simulink model "VFlexP_small"  (R2026a)
settings: Solver=ode23tb  StopTime=2  FixedStep=5e-5
model workspace (MAT data in the model file):
  DCop_DCBUCK : object (value not decoded)
  Grid_CCVSC_idx = [2; 3; 4; 5; 6; 7; 8; 9; 10; 11; 12]
  Grid_CCVSCs = 1
  Grid_CCVSCs_buses = 1
  Grid_CCVSCs_toM = [0 1 0 0 0 0 0 0 0 0 0 0 ... (781 elements, 71x11)]
  Grid_C_Lines = 0
  Grid_Cbuses = [0.00666666666667 0.00666666666667]
  Grid_DC : object (value not decoded)
  Grid_DCop_DCBUCK : object (value not decoded)
  Grid_DCop_DC_PES : object (value not decoded)
  Grid_DFIGs = 1
  Grid_DFIGs_buses = 1
  Grid_DGs : string (value not decoded)
  Grid_From_buses = 1
  Grid_GFls = 1
  Grid_GFls_buses = 1
  Grid_GFr_idx = 1
  Grid_GFrs = 1
  Grid_GFrs_buses = 1
  Grid_GFrs_toM = [1; 0]
  Grid_IG_idx = 1
  Grid_IGs = 1
  Grid_IGs_buses = 1
  Grid_IGs_toM = [1; 0; 0]
  Grid_L_Lines = 0.05
  Grid_L_Loads = [0 0]
  Grid_Lines_fromM : object (value not decoded)
  Grid_Lines_toM : object (value not decoded)
  Grid_Load_buses = [1; 2]
  Grid_Load_busesDC = []
  Grid_MSGs = 1
  Grid_MSGs_buses = 1
  Grid_Nbuses = 2
  Grid_PQ_gen = 3
  Grid_Ploads = [0.0075 0.0075]
  Grid_PloadsDC = []
  Grid_Ps_lf = 0.51232912
  Grid_Qloads = [0 0]
  Grid_Qs_lf = -0.00723209333333
  Grid_R_Lines = 0.005
  Grid_R_Loads = [2 2]
  Grid_R_Loads_DC = 0
  Grid_Rcf = [150 150]
  Grid_SCs = 1
  Grid_SCs_buses = 1
  Grid_SG_idx = 1
  Grid_SGs = 1
  Grid_SGs_buses = 1
  Grid_SGs_toM = [1; 0]
  Grid_To_buses = 2
  Grid_VCVSC_idx = [1; 2; 3; 4; 5; 6; 7; 8; 9; 10; 11; 12]
  Grid_VCVSCs = 1
  Grid_VCVSCs_buses = [1; 2; 3; 6; 8; 9; 12; 58; 59; 60; 63; 65]
  Grid_VCVSCs_toM = [1 0 0 0 0 0 0 0 0 0 0 0 ... (852 elements, 71x12)]
  Grid_VSM_idx = 2
  Grid_VSMs = 1
  Grid_VSMs_buses = 1
  Grid_VSMs_toM = [0; 1]
  Grid_admitt_matrix = [2.15353135314-19.7953135314i  -1.9801980198+19.801980198i; -1.9801980198+19.801980198i  2.15353135314-19.7953135314i]
  Grid_admitt_matrix_noloads = [1.98686468647-19.7953135314i  -1.9801980198+19.801980198i; -1.9801980198+19.801980198i  1.98686468647-19.7953135314i]
  Grid_bus = [1; 2]
  Grid_busDC_complexity = 1
  Grid_busDC_complexity_PF = 2
  Grid_bus_complexity = [1 1]
  Grid_bus_complexity_PF = [1 1]
  Grid_buses_lf = 1
  Grid_conductance_matrix = 0.00666666666667
  Grid_conductance_matrix_noloads = 0.00666666666667
  Grid_fref : object (value not decoded)
  Grid_gen_static_params : mBase (value not decoded)
  Grid_iPs_lf = 1.95187031336
  Grid_iQs_lf = -138.272551792
  Grid_iadmitt_matrix = [2.88165849328-0.0982918688642i  2.87905051706-0.123273862303i; 2.87905051706-0.123273862303i  2.88165849328-0.0982918688642i]
  Grid_iadmitt_matrix_noloads = [37.5012524798-37.4874983544i  37.4987475202-37.5125016456i; 37.4987475202-37.5125016456i  37.5012524798-37.4874983544i]
  Grid_iconductance_matrix = 150
  Grid_iconductance_matrix_noloads = 150
  Grid_init_OK_bool = 1
  Grid_intconv_PF : object (value not decoded)
  Grid_lf_op : op_report (value not decoded)
  Grid_lineDC_complexity = []
  Grid_lineDC_complexity_PF = []
  Grid_line_complexity = 1
  Grid_line_complexity_PF = 3
  Grid_loadDC_complexity = []
  Grid_loadDC_complexity_PF = []
  Grid_load_complexity = [3 3]
  Grid_load_complexity_PF = [4 4]
  Grid_opDC_CCVSC : object (value not decoded)
  Grid_opDC_VSM : object (value not decoded)
  Grid_opGFr : object (value not decoded)
  Grid_opVCVSC : object (value not decoded)
  Grid_op_CCVSC : object (value not decoded)
  Grid_op_IG : object (value not decoded)
  Grid_op_SG : object (value not decoded)
  Grid_op_VSM : object (value not decoded)
  Grid_shift_lines = 0
  Grid_tap_lines = 1
  Grid_v_buses_mod = [1 1]
  LinsysParamChangeStruct : Param1 (value not decoded)
  Lline = 0.01
  Rline = 1e-05
  linsys : object (value not decoded)
values from neighbouring files (symbols this model uses):
  block_idx = evalin(mdlWks, [bvarname Generators{i} '_idx'])    [fun_init_units_callback.m]
  Fb = areas    [fun_MATPOWER_to_Excel.m]
  Fi = evalin('base', get_param(block, 'Fi'))    [fun_init_GFr.m]    (also in fun_init_intconv_DC_VSM.m)
  Lf = evalin('base', get_param(block, 'Lf'))    [fun_init_GFr.m]    (also in fun_init_intconv_DC_VSM.m)
  Rf = evalin('base', get_param(block, 'Rf'))    [fun_init_GFr.m]    (also in fun_init_intconv_DC_VSM.m)
symbols that are objects in the model workspace (value not decoded): Grid_DCop_DC_PES, Grid_DCop_DCBUCK, Grid_op_CCVSC, Grid_op_IG, Grid_op_SG, Grid_op_VSM, Grid_opDC_CCVSC, Grid_opDC_VSM, Grid_opGFr, Grid_opVCVSC
undefined symbols (not defined in the file or in its folder): block_buses_DC, CCVSC_idx, Cf, costs, costs2, DFIGs_nodes, DiscIntNeverNeededParam, entity, From_nodes, grid_linsys, Grid_op_DFIG, Grid_op_DFIG_PQ, Grid_op_MSG, Grid_op_SC, Grid_op_VCVSC, Hv, initial_states_grid, Kic, Kiv, Kp_theta, Kp_w, Kpc, Kpv, last_send, Lc, m, Matrix_flux_to_i, mD, mp, MSGs_buses, Nbuses_DC, nq, op_VCVSC, Psche, Rc, rkq1, rkq2, SCs_buses, SCs_nodes, sec_control_structure, set_asked, set_DG_up, set_extra_satur, set_sending_cost, SGs_buses, SGs_nodes, Tf, To_nodes, VI_L, VI_R, WOF_Tf, xkq1, xkq2
libraries: simulink x1045, eeGeneralControl x12, eeTransforms x1, sl_discontinuities x1
(part 8 of 50)

== system VFlexP_small/Grid/Dynamic/Secondary Control/Matrices1 ==
  tertiary_refs : Inport
  start_SC : Inport  Port=2
  elec : Inport  Port=3
  Assignment{,1..2,13} (4 alike) : Assignment  NumberOfDimensions=2  DiagnosticForDimensions=Warning  IndexOptions=Index vector (dialog),Assign all  Indices=2,1  OutputSizes=1,1
  Assignment10 : Assignment  NumberOfDimensions=2  DiagnosticForDimensions=Warning  IndexOptions=Index vector (dialog),Assign all  Indices=1,1  OutputSizes=1,1
  Assignment{3..4,9,11} (4 alike) : Assignment  DiagnosticForDimensions=Warning  IndexOptions=Index vector (port)  Indices=1  OutputSizes=1
  Assignment12 : Assignment  NumberOfDimensions=2  DiagnosticForDimensions=Warning  IndexOptions=Index vector (dialog),Assign all  Indices=1,1  OutputSizes=1,1
  Assignment{5..8} (4 alike) : Assignment  NumberOfDimensions=2  DiagnosticForDimensions=Warning  IndexOptions=Index vector (port),Assign all  Indices=1,1  OutputSizes=1,1
  Cast To Double1 : DataTypeConversion  OutDataTypeStr=double  SaturateOnIntegerOverflow=off  RndMeth=Floor
  Compare To Constant : simulink/Logic and Bit Operations/Compare To Constant  relop=>  const=0.8  OutDataTypeStr=boolean
  Compare To Constant1 : simulink/Logic and Bit Operations/Compare To Constant  relop=<  const=0  OutDataTypeStr=boolean
  Compare To Constant2 : simulink/Logic and Bit Operations/Compare To Constant  relop=>  const=3  OutDataTypeStr=boolean
  Constant : Constant  Commented=on  Value=costs'  VectorParams1D=off
  Constant1 : Constant  Commented=on  Value=2*costs2'  VectorParams1D=off
  Constant10 : Constant  Value=A_P_sc  VectorParams1D=off
  Constant11 : Constant  Value=A_v_sc  VectorParams1D=off
  Constant12 : Constant  Value=A_Q_sc  VectorParams1D=off
  Constant13 : Constant
  Constant14 : Constant  Value=0
  Constant15 : Constant  Value=zeros(1, length(buses_lf))  VectorParams1D=off
  Constant16 : Constant  Commented=on  Value=sec_control_structure
  Constant18 : Constant  Commented=on  Value=sec_control_structure
  Constant19 : Constant  Commented=on  VectorParams1D=off
  Constant2 : Constant  Value=repmat([1 1 1 1]', 1, length(buses_lf))
  Constant20 : Constant  Value=passM  VectorParams1D=off
  Constant3 : Constant  Commented=on
  Constant4 : Constant  Value=length(buses_lf)
  Constant5 : Constant  Value=g_f_sc'  VectorParams1D=off
  Constant6 : Constant  Value=g_P_sc'  VectorParams1D=off
  Constant7 : Constant  Value=g_v_sc'  VectorParams1D=off
  Constant8 : Constant  Value=g_Q_sc'  VectorParams1D=off
  Constant9 : Constant  Value=A_f_sc  VectorParams1D=off
  Display{,1..9} (10 alike) : Display
  Divide : Product  Commented=on  Inputs=*/
  Gain1 : Gain  Commented=on  Gain=1/400
  Gain11 : Gain  Commented=on  Gain=1/400
  Gain2 : Gain  Gain=20
  Gain9 : Gain  Gain=-1
  Integrator : Integrator
  Integrator1 : Integrator  ExternalReset=rising
  Matrix Concatenate : Concatenate  NumInputs=4  Mode=Multidimensional array
  Matrix Concatenate1 : Concatenate  NumInputs=3  Mode=Multidimensional array
  Matrix Concatenate2 : Concatenate  NumInputs=4  Mode=Multidimensional array
  Matrix Multiply{,1..4} (5 alike) : Product  Multiplication=Matrix(*)
  Memory1 : Memory
  Memory2 : Memory  InitialCondition=1
  Mod : Math  Operator=mod
  Multiport Switch : MultiPortSwitch  Commented=on  Inputs=5  SaturateOnIntegerOverflow=off  InputSameDT=off
  NOT : Logic  Operator=NOT  IconShape=distinctive  AllPortsSameDT=off  OutDataTypeStr=boolean
  OR1 : Logic  Operator=OR  Inputs=3  IconShape=distinctive  AllPortsSameDT=off  OutDataTypeStr=boolean
  One : Constant  OutDataTypeStr=Inherit: Inherit via back propagation
  One1 : Constant  OutDataTypeStr=Inherit: Inherit via back propagation
  One3 : Constant  Commented=on  OutDataTypeStr=Inherit: Inherit via back propagation
  Product{,2..4,7,9..12} (9 alike) : Product
  Product1 : Product  Commented=on
  Product13 : Product  Commented=on
  Product14 : Product  Commented=on
  Relational Operator : RelationalOperator  Operator===  OutDataTypeStr=boolean  RndMeth=Simplest  InputSameDT=off
  Relational Operator1 : RelationalOperator  Operator===  OutDataTypeStr=boolean  RndMeth=Simplest  InputSameDT=off
  Selector{,9,19,22,26,28} (6 alike) : Selector  NumberOfDimensions=2  InputPortWidth=3  IndexOptions=Index vector (dialog),Select all  Indices=1,1  OutputSizes=1,1
  Selector{1,7,10,13..15,20..21,23..25,27} (12 alike) : Selector  NumberOfDimensions=2  InputPortWidth=3  IndexOptions=Index vector (dialog),Select all  Indices=2,1  OutputSizes=1,1
  Selector11 : Selector  NumberOfDimensions=2  InputPortWidth=3  IndexOptions=Index vector (dialog),Select all  Indices=4,1  OutputSizes=1,1
  Selector12 : Selector  NumberOfDimensions=2  InputPortWidth=length(buses_lf)  IndexOptions=Index vector (dialog),Index vector (port)  Indices=6,1  OutputSizes=1,1
  Selector16 : Selector  NumberOfDimensions=2  InputPortWidth=length(buses_lf)  IndexOptions=Index vector (dialog),Index vector (port)  Indices=2,1  OutputSizes=1,1
  Selector17 : Selector  NumberOfDimensions=2  InputPortWidth=3  IndexOptions=Index vector (dialog),Index vector (port)  Indices=1,1  OutputSizes=1,1
  Selector18 : Selector  Commented=on  NumberOfDimensions=2  InputPortWidth=3  IndexOptions=Index vector (dialog),Select all  Indices=2,1  OutputSizes=1,1
  Selector2 : Selector  NumberOfDimensions=2  InputPortWidth=3  IndexOptions=Index vector (dialog),Select all  Indices=3,1  OutputSizes=1,1
  Selector3 : Selector  NumberOfDimensions=2  InputPortWidth=3  IndexOptions=Index vector (dialog),Select all  Indices=4,1  OutputSizes=1,1
  Selector4 : Selector  NumberOfDimensions=2  InputPortWidth=3  IndexOptions=Index vector (dialog),Select all  Indices=5,1  OutputSizes=1,1
  Selector5 : Selector  NumberOfDimensions=2  InputPortWidth=3  IndexOptions=Index vector (dialog),Select all  Indices=6,1  OutputSizes=1,1
  Selector6 : Selector  NumberOfDimensions=2  InputPortWidth=3  IndexOptions=Index vector (dialog),Select all  Indices=1:4,1  OutputSizes=1,1
  Selector8 : Selector  NumberOfDimensions=2  InputPortWidth=3  IndexOptions=Index vector (dialog),Select all  Indices=3,1  OutputSizes=1,1
  Sum{,1..3,5,9,11} (7 alike) : Sum  Inputs=|++
  Sum of Elements{,1..3} (4 alike) : Sum  Inputs=+  CollapseMode=Specified dimension  CollapseDim=2
  Sum10 : Sum  Inputs=|+-
  Sum4 : Sum  Inputs=|-+
  Sum6 : Sum  Inputs=|+-
  Sum7 : Sum  Commented=on  Inputs=|++
  Switch : Switch  Criteria=u2 > Threshold  SaturateOnIntegerOverflow=off  InputSameDT=off
  Switch1 : Switch  Criteria=u2 > Threshold  SaturateOnIntegerOverflow=off  InputSameDT=off
  Switch2 : Switch  Commented=on  Criteria=u2 > Threshold  SaturateOnIntegerOverflow=off  InputSameDT=off
  Switch3 : Switch  Commented=on  Criteria=u2 > Threshold  Threshold=1  SaturateOnIntegerOverflow=off  InputSameDT=off
  Transport Delay : TransportDelay  DelayTime=0.1  PadeOrder=3
  Transpose{,1..17} (18 alike) : Math  Operator=transpose
  Triggered Subsystem : Subsystem  TreatAsAtomicUnit=on
  Zero : Constant  Value=zeros(1, length(buses_lf))  VectorParams1D=off  OutDataTypeStr=Inherit: Inherit via back propagation
  Zero1 : Constant  Value=zeros(1, length(buses_lf))  VectorParams1D=off  OutDataTypeStr=Inherit: Inherit via back propagation
  Zero2 : Constant  Value=zeros(1, length(buses_lf))  VectorParams1D=off  OutDataTypeStr=Inherit: Inherit via back propagation
  saturation_P : Subsystem
  saturation_P2 : Subsystem
  start_SC1 : InportShadow  Port=2
  secondary_refs : Outport
  wires:
  Selector3/1 -> Transpose3/1  "Q"
  Selector/1 -> Transpose/1  "f"
  Selector1/1 -> Product2/1, Transpose13/1  "P"
  Selector2/1 -> Transpose2/1  "v"
  Sum/1 -> Transpose4/1
  Product9/1 -> Sum/2
  Product10/1 -> Sum1/2
  Matrix Multiply2/1 -> Sum2/1
  Product11/1 -> Sum2/2
  Product12/1 -> Sum3/2
  Sum2/1 -> Transpose6/1
  Sum3/1 -> Transpose7/1
  Matrix Multiply3/1 -> Sum3/1
  Transpose/1 -> Matrix Multiply/2
  Transpose1/1 -> Matrix Multiply1/2
  Transpose2/1 -> Matrix Multiply2/2
  Transpose3/1 -> Matrix Multiply3/2
  Transpose6/1 -> Matrix Concatenate/3
  Transpose7/1 -> Matrix Concatenate/4
  Selector8/1 -> Transpose10/1
  Selector4/1 -> Matrix Concatenate1/2
  start_SC/1 -> Switch/2
  Switch/1 -> secondary_refs/1, Selector19/1, Selector15/1
  Selector5/1 -> Matrix Concatenate1/3
  Selector9/1 -> Transpose8/1
  Selector10/1 -> Transpose9/1
  Selector11/1 -> Transpose11/1
  Sum5/1 -> Switch/1
  Transpose8/1 -> Product9/2
  Transpose9/1 -> Product10/2
  Transpose10/1 -> Product11/2
  Transpose11/1 -> Product12/2
  Matrix Concatenate/1 -> Sum6/1
  start_SC1/1 -> Product/2
  Transport Delay/1 -> Selector2/1, Selector3/1, Selector1/1, Selector/1, Gain9/1
  Constant1/1 -> Product1/1
  Product2/1 -> Transpose1/1
  [gaincost] -> Product2/2
  Product7/1 -> Assignment/1, Selector7/1
  [gaincost] -> Product3/2
  Selector7/1 -> Product3/1
  Assignment/1 -> Sum6/2, Selector24/1
  saturation_P/1(out) -> Matrix Concatenate/2, Relational Operator/1
  Product3/1 -> Assignment/2
  Selector13/1 -> [Pref]
  Selector14/1 -> Switch2/2, Switch1/1
  Switch1/1 -> Assignment2/2
  Transpose4/1 -> Matrix Concatenate/1
  Matrix Multiply1/1 -> Sum1/1
  Matrix Multiply/1 -> Sum/1
  Sum of Elements/1 -> Transpose14/1
  Sum of Elements1/1 -> Transpose15/1
  Sum of Elements2/1 -> Transpose16/1
  Sum of Elements3/1 -> Transpose17/1
  Transpose17/1 -> Matrix Concatenate2/4
  Transpose16/1 -> Matrix Concatenate2/3
  Transpose14/1 -> Matrix Concatenate2/2
  Transpose15/1 -> Matrix Concatenate2/1
  Selector6/1 -> Product7/1
  Matrix Concatenate2/1 -> Product7/2
  [A_f_sc] -> Sum of Elements1/1
  [A_P_sc] -> Sum of Elements/1
  [A_Q_sc] -> Sum of Elements3/1
  [A_v_sc] -> Sum of Elements2/1
  [A_f_sc] -> Matrix Multiply/1
  [A_P_sc] -> Matrix Multiply1/1
  [A_v_sc] -> Matrix Multiply2/1
  [A_Q_sc] -> Matrix Multiply3/1
  [g_f_sc] -> Product9/1
  [g_v_sc] -> Product11/1
  [g_Q_sc] -> Product12/1
  [g_P_sc] -> Product10/1
  Constant5/1 -> Assignment3/1
  Constant13/1 -> Assignment4/2, Assignment3/2
  [leader] -> Assignment4/3, Assignment3/3
  Constant6/1 -> [g_P_sc]
  Constant8/1 -> [g_Q_sc]
  Constant7/1 -> Assignment4/1
  Constant9/1 -> Assignment5/1
  Constant12/1 -> Assignment8/1
  Constant11/1 -> Assignment7/1
  Constant10/1 -> Assignment6/1
  [leader] -> Assignment9/3
  [leader] -> Assignment5/3, Assignment6/3, Assignment7/3, Assignment8/3
  Constant14/1 -> Assignment9/2
  Zero/1 -> Assignment9/1
  Assignment9/1 -> Assignment8/2, Assignment6/2
  Zero1/1 -> Assignment7/2, Assignment5/2
  Memory2/1 -> Selector12/2, Sum10/1, Selector16/2
  elec/1 -> Selector18/1, Selector12/1, Selector16/1, Sum4/2
  Selector16/1 -> Compare To Constant1/1, Compare To Constant/1
  Cast To Double1/1 -> Integrator1/1
  Mod/1 -> Sum9/1
  One/1 -> Sum9/2
  Triggered Subsystem/1(Out1) -> Mod/1
  Constant4/1 -> Mod/2
  [leader] -> Memory2/1
  Compare To Constant/1 -> OR1/1
  Compare To Constant1/1 -> OR1/2
  [leader] -> Assignment11/3, Selector17/2
  Selector17/1 -> Assignment11/2
  Constant15/1 -> Assignment11/1
  Integrator1/1 -> Compare To Constant2/1
  Compare To Constant2/1 -> Memory1/1, Triggered Subsystem/Trigger
  OR1/1 -> Cast To Double1/1
  Memory1/1 -> Integrator1/2
  Sum7/1 -> Gain11/1
  Gain11/1 -> Multiport Switch/5, Product13/2, Product13/1
  Product1/1 -> Sum7/2
  Selector18/1 -> Product1/2
  Constant3/1 -> [gaincost], Multiport Switch/2
  Constant16/1 -> Multiport Switch/1
  Sum10/1 -> Triggered Subsystem/1(In1)
  One1/1 -> Sum10/2
  Matrix Concatenate1/1 -> Sum5/1
  Constant/1 -> Gain1/1, Sum7/1
  Gain1/1 -> Multiport Switch/3, Product14/2, Product14/1
  Product14/1 -> Multiport Switch/4
  Product13/1 -> Multiport Switch/6
  Multiport Switch/1 -> Divide/2, Switch2/1
  Constant18/1 -> Switch3/2
  Divide/1 -> Switch3/1
  One3/1 -> Switch3/3
  Constant19/1 -> Divide/1
  tertiary_refs/1 -> Sum4/1, Selector13/1, Selector4/1, Selector5/1, Switch/3, Sum5/2
  Constant20/1 -> Matrix Multiply4/1
  Matrix Multiply4/1 -> Transpose12/1
  [awup1] -> Switch1/2
  Transpose13/1 -> Matrix Multiply4/2
  Switch3/1 -> Switch2/3
  Sum9/1 -> [leader]
  Gain9/1 -> Selector11/1, Selector8/1, Selector10/1, Selector9/1
  Sum6/1 -> Product4/1
  Assignment11/1 -> Assignment10/2
  [gaincost] -> saturation_P/3(gaincost)
  Transpose5/1 -> saturation_P/2(in), Relational Operator/2
  [Pref] -> saturation_P/1(Pref)
  Relational Operator/1 -> [awup1]
  Assignment2/1 -> Transport Delay/1
  Selector12/1 -> NOT/1
  NOT/1 -> OR1/3
  Selector15/1 -> Display/1
  Selector19/1 -> Display1/1
  Sum1/1 -> Transpose5/1
  Zero2/1 -> Assignment12/2
  Assignment12/1 -> Matrix Concatenate1/1
  Selector22/1 -> Gain2/1
  Gain2/1 -> Sum11/1
  Product/1 -> Assignment13/1, Selector22/1, Selector23/1
  Selector23/1 -> Sum11/2
  Selector20/1 -> Display2/1
  Sum4/1 -> Selector20/1, Assignment2/1, Selector14/1, Selector6/1
  Sum11/1 -> Assignment13/2
  saturation_P2/1(out) -> Assignment1/2, Relational Operator1/2, Display8/1
  Relational Operator1/1 -> [awup2]
  Selector21/1 -> Display9/1, Relational Operator1/1, saturation_P2/2(in)
  [Pref] -> saturation_P2/1(Pref)
  Assignment1/1 -> Assignment12/1
  Constant2/1 -> Product4/2
  Assignment3/1 -> [g_f_sc]
  Assignment4/1 -> [g_v_sc]
  Transpose12/1 -> Switch1/3
  Selector24/1 -> Display3/1
  Product4/1 -> Product/1
  [A_P_sc] -> saturation_P/4(A_P_SC)
  Selector25/1 -> Display4/1
  Assignment13/1 -> Selector26/1, Selector25/1, Integrator/1
  Selector26/1 -> Display5/1
  Selector28/1 -> Display7/1
  Integrator/1 -> Selector27/1, Selector28/1, Assignment1/1, Selector21/1
  Selector27/1 -> Display6/1
  Assignment5/1 -> [A_f_sc]
  Assignment6/1 -> [A_P_sc]
  Assignment7/1 -> [A_v_sc]
  Assignment8/1 -> [A_Q_sc]

== system VFlexP_small/Grid/Dynamic/Secondary Control/No SC ==
  tertiary_refs : Inport
  secondary_refs : Outport
  wires:
  tertiary_refs/1 -> secondary_refs/1

== system VFlexP_small/Grid/Dynamic/Secondary Control/Pilot nodes ==
  tertiary_refs : Inport
  start_SC : Inport  Port=2
  v_buses : Inport  Port=3
  Complex to Magnitude-Angle : ComplexToMagnitudeAngle  Output=Magnitude
  Gain : Gain  Gain=-1
  I1 : Integrator
  Matrix Concatenate : Concatenate  NumInputs=6  Mode=Multidimensional array
  One : Constant  OutDataTypeStr=Inherit: Inherit via back propagation
  PI : Subsystem
  PI1 : Subsystem
  PLL : Subsystem
  Product : Product
  Product1 : Product
  Product2 : Product
  Real-Imag to Complex : RealImagToComplex
  Reference frame transform3 : Subsystem
  Selector1 : Selector  NumberOfDimensions=2  InputPortWidth=3  IndexOptions=Index vector (dialog),Select all  Indices=2,1  OutputSizes=1,1
  Selector10 : Selector  InputPortWidth=length(fref.ref_units)  IndexOptions=Index vector (dialog)  Indices=fref.Fb_units  OutputSizes=1
  Selector12 : Selector  NumberOfDimensions=2  InputPortWidth=3  IndexOptions=Index vector (dialog),Select all  Indices=3,1  OutputSizes=1,1
  Selector2 : Selector  NumberOfDimensions=2  InputPortWidth=3  IndexOptions=Index vector (dialog),Select all  Indices=3,1  OutputSizes=1,1
  Selector3 : Selector  NumberOfDimensions=2  InputPortWidth=3  IndexOptions=Index vector (dialog),Select all  Indices=4,1  OutputSizes=1,1
  Selector4 : Selector  NumberOfDimensions=2  InputPortWidth=3  IndexOptions=Index vector (dialog),Select all  Indices=5,1  OutputSizes=1,1
  Selector5 : Selector  NumberOfDimensions=2  InputPortWidth=3  IndexOptions=Index vector (dialog),Index vector (dialog)  Indices=2,buses_lf  OutputSizes=1,1
  Selector6 : Selector  NumberOfDimensions=2  InputPortWidth=3  IndexOptions=Index vector (dialog),Index vector (dialog)  Indices=1,buses_lf  OutputSizes=1,1
  Selector7 : Selector  NumberOfDimensions=2  InputPortWidth=3  IndexOptions=Index vector (dialog),Select all  Indices=1,1  OutputSizes=1,1
  Selector8 : Selector  NumberOfDimensions=2  InputPortWidth=3  IndexOptions=Index vector (dialog),Select all  Indices=6,1  OutputSizes=1,1
  Selector9 : Selector  InputPortWidth=length(fref.ref_units)  IndexOptions=Index vector (dialog)  Indices=fref.Fb_units  OutputSizes=1
  Sum : Sum  Inputs=|++
  Sum1 : Sum  Inputs=|+-
  Sum2 : Sum  Inputs=|+-
  Sum3 : Sum  Inputs=|++
  Sum4 : Sum  Inputs=|+-
  Switch : Switch  Criteria=u2 > Threshold  SaturateOnIntegerOverflow=off  InputSameDT=off
  start_SC1 : InportShadow  Port=2
  secondary_refs : Outport
  wires:
  Sum/1 -> Matrix Concatenate/4
  Matrix Concatenate/1 -> Switch/1
  Selector3/1 -> Sum/1
  Selector1/1 -> Matrix Concatenate/2
  Selector2/1 -> Matrix Concatenate/3
  Selector4/1 -> Matrix Concatenate/5
  start_SC/1 -> Switch/2
  Switch/1 -> secondary_refs/1
  tertiary_refs/1 -> Selector12/1, Selector7/1, Selector1/1, Selector2/1, Switch/3, Selector3/1, Selector8/1, Selector4/1
  Product/1 -> PI/1(Input)
  Sum3/1 -> Matrix Concatenate/1  "f"
  Selector8/1 -> Matrix Concatenate/6
  start_SC1/1 -> Product/2, Product1/2
  Product1/1 -> PI1/1(Input)
  Sum2/1 -> Product2/1  "omega2"
  Selector5/1 -> Reference frame transform3/3(in_q)
  v_buses/1 -> Selector5/1, Selector6/1
  Selector6/1 -> Reference frame transform3/1(in_d)
  Reference frame transform3/2(out_q) -> PLL/1(out_q), Real-Imag to Complex/2
  Product2/1 -> I1/1
  I1/1 -> Gain/1
  One/1 -> Sum1/1
  PLL/1(Input2) -> Sum1/2, Sum2/1  "omega2"
  Selector9/1 -> Sum2/2
  Gain/1 -> Reference frame transform3/2(theta)
  Sum1/1 -> Product1/1
  Selector7/1 -> Sum3/1
  PI1/1(Out1) -> Sum3/2  "f"
  [omega_ref] -> Selector9/1
  Selector10/1 -> Product2/2
  [omega_base] -> Selector10/1
  PI/1(Out1) -> Sum/2
  Selector12/1 -> Sum4/1
  Complex to Magnitude-Angle/1 -> Sum4/2
  Reference frame transform3/1(out_d) -> Real-Imag to Complex/1  "v CCVSC"
  Real-Imag to Complex/1 -> Complex to Magnitude-Angle/1
  Sum4/1 -> Product/1

== system VFlexP_small/Grid/Dynamic/Tertiary Control/MAS edp ==
  elec : Inport
  connect_DGs : Inport  Port=2
  Clock : Clock
  Compare To Constant : simulink/Logic and Bit Operations/Compare To Constant  relop=>  const=150  OutDataTypeStr=boolean
  Constant : Constant  Value=[ones(1, length(buses_lf)); Ps_lf; v_buses_mod(buses_lf); Qs_lf]  VectorParams1D=off
  Matrix Concatenate1 : Concatenate  NumInputs=6  Mode=Multidimensional array
  Matrix Concatenate2 : Concatenate  NumInputs=3  Mode=Multidimensional array
  One : Constant  Value=v_buses_mod(buses_lf)  VectorParams1D=off  OutDataTypeStr=Inherit: Inherit via back propagation
  One1 : Constant  Value=Qs_lf  VectorParams1D=off  OutDataTypeStr=Inherit: Inherit via back propagation
  One2 : Constant  Value=ones(1, length(buses_lf))  VectorParams1D=off  OutDataTypeStr=Inherit: Inherit via back propagation
  Pmax : Constant  Value=max(0.03*ones(1, length(Ps_lf)), Ps_lf)  VectorParams1D=off
  Pmin : Constant  Value=min(0*ones(1, length(Ps_lf)), Ps_lf*0.5)  VectorParams1D=off
  Pulse Generator : DiscretePulseGenerator  PulseType=Time based  Period=100  PulseWidth=5  PhaseDelay=2
  Selector1 : Selector  NumberOfDimensions=2  InputPortWidth=3  IndexOptions=Index vector (dialog),Select all  Indices=6,1  OutputSizes=1,1
  Selector2 : Selector  NumberOfDimensions=2  InputPortWidth=3  IndexOptions=Index vector (dialog),Select all  Indices=2,1  OutputSizes=1,1
  Selector6 : Selector  NumberOfDimensions=2  InputPortWidth=3  IndexOptions=Index vector (dialog),Select all  Indices=6,1  OutputSizes=1,1
  Subsystem : Subsystem  mask{A=circshift(eye(length(buses_lf)), -1), gainM=0.001}
      settings: PortSchema="{\"entries\":[{\"content\":{\"sides\":[{\"content\":{\"connectorIds\":[\"In1\",\"In2\",\"In3\",\"In4\",\"In5\"]},\"type\":\"ConnectorPlacement.EquallySpacedRectSide\",\"uuid\":\"cdca2cdc-0a32-4006-9eb7-95eef3e074c5\"},{\"content\":{\"connectorIds\":[\"Out1\"],\"side\":\"RIGHT\"},\"type\":\"ConnectorPlacement.EquallySpacedRectSide\",\"uuid\":\"477e4c44-ed13-4581-bb25-eee9ea5698cb\"},{\"content\":{\"connectorIds\":[\"In6\"],\"side\":\"TOP\"},\"type\":\"ConnectorPlacement.EquallySpacedRectSide\",\"uuid\":\"390c7fbe-2640-4698-bec4-03c3001b65dc\"}]},\"type\":\"ConnectorPlacement.EquallySpacedConnector\",\"uuid\":\"648f22ad-3aa2-45b0-803b-7637b6161fb1\"}],\"packageUris\":[\"http://schema.mathworks.com/mf0/Connector/R2020b\"],\"version\":\"1.0\"}"
  Switch : Switch  Criteria=u2 > Threshold  SaturateOnIntegerOverflow=off  InputSameDT=off
  Transpose{,1..3} (4 alike) : Math  Operator=transpose
  costs : UniformRandomNumber  Minimum=0  Seed=(1:length(buses_lf))'  SampleTime=100  VectorParams1D=off
  costs2 : UniformRandomNumber  Minimum=0  Seed=9*(1:length(buses_lf))'  SampleTime=100  VectorParams1D=off
  ref : Outport
  wires:
  Clock/1 -> Compare To Constant/1
  Compare To Constant/1 -> Switch/2
  One/1 -> Matrix Concatenate1/3
  Matrix Concatenate1/1 -> Switch/1
  Pmin/1 -> Transpose2/1
  Pmax/1 -> Transpose1/1
  One1/1 -> Matrix Concatenate1/4
  One2/1 -> Matrix Concatenate1/1
  [connect] -> Matrix Concatenate1/5
  Selector1/1 -> Matrix Concatenate1/6
  [connect] -> Matrix Concatenate2/2
  Selector6/1 -> Matrix Concatenate2/3
  Constant/1 -> Matrix Concatenate2/1
  Switch/1 -> ref/1
  Matrix Concatenate2/1 -> Switch/3
  connect_DGs/1 -> [connect]
  elec/1 -> Selector6/1, Selector1/1, Selector2/1
  Subsystem/1(Pref) -> Transpose3/1
  costs/1 -> Subsystem/1(costs)
  costs2/1 -> Subsystem/2(costs2)
  Selector2/1 -> Transpose/1
  Transpose/1 -> [x0]
  Pulse Generator/1 -> Subsystem/6(start)
  [x0] -> Subsystem/5(x0)
  Transpose1/1 -> Subsystem/3(Pmax)
  Transpose2/1 -> Subsystem/4(Pmin)
  Transpose3/1 -> Matrix Concatenate1/2

== system VFlexP_small/Grid/Dynamic/Tertiary Control/MAS messages ==
  elec : Inport
  Constant1 : Constant  Value=1000*ones(1, length(buses_lf))  VectorParams1D=off
  Constant2 : Constant  Value=100*ones(1, length(buses_lf))  VectorParams1D=off
  Costs : RandomNumber  Mean=2*ones(1,length(buses_lf))  Variance=1*ones(1,length(buses_lf))  Seed=1:length(buses_lf)  SampleTime=100  VectorParams1D=off
  Goto Tag Visibility : GotoTagVisibility  GotoTag=Pmax
  Goto Tag Visibility1 : GotoTagVisibility  GotoTag=Snom
  Goto Tag Visibility2 : GotoTagVisibility  GotoTag=costs
  ID1 : Subsystem  VariantControl=multi-agent  mask(gen_agent){ID=1, Leader=Leader, NeighN=2, Neigh1=7, Neigh2=2, Neigh3=0, Neigh4=0, Neigh5=0}
      mask prompts: ID "ID number"; Leader "Leader multi-agent"; NeighN "Number of neighbors"; Neigh1 "Neighbor 1"; Neigh2 "Neighbor 2"; Neigh3 "Neighbor 3"; Neigh4 "Neighbor 4"; Neigh5 "Neighbor 5"
      mask init: same as VFlexP_small/Grid/Dynamic/Secondary Control/MAS messages/ID1
      mask TypeOptions Leader: No leader | Leader
      mask TypeOptions NeighN: 1 | 2 | 3 | 4 | 5
      mask Callback NeighN:
      | block = gcb;
      | NeighN = str2double(get_param(block, 'NeighN'));
      | param_vis = get_param(block,'MaskVisibilities');
      | block_params = string(fieldnames(get_param(block, 'DialogParameters')));
      | param_vis(find(block_params == 'Neigh1'):find(block_params == 'Neigh5')) = cellstr("on");
      | if NeighN < 5 % Hide some
      |     param_vis(find(block_params == 'Neigh1')+NeighN:find(block_params == 'Neigh5')) = cellstr("off");
      | end
      | set_param(block,'MaskVisibilities',param_vis)
      mask DialogControl Container8 Prompt: Parameters
  ID2 : Subsystem  VariantControl=multi-agent  mask(gen_agent){ID=2, Leader=No leader, NeighN=2, Neigh1=1, Neigh2=3, Neigh3=0, Neigh4=0, Neigh5=0}
      mask prompts: ID "ID number"; Leader "Leader multi-agent"; NeighN "Number of neighbors"; Neigh1 "Neighbor 1"; Neigh2 "Neighbor 2"; Neigh3 "Neighbor 3"; Neigh4 "Neighbor 4"; Neigh5 "Neighbor 5"
      mask init: same as VFlexP_small/Grid/Dynamic/Secondary Control/MAS messages/ID1
      mask TypeOptions Leader: No leader | Leader
      mask TypeOptions NeighN: 1 | 2 | 3 | 4 | 5
      mask Callback NeighN:
      | block = gcb;
      | NeighN = str2double(get_param(block, 'NeighN'));
      | param_vis = get_param(block,'MaskVisibilities');
      | block_params = string(fieldnames(get_param(block, 'DialogParameters')));
      | param_vis(find(block_params == 'Neigh1'):find(block_params == 'Neigh5')) = cellstr("on");
      | if NeighN < 5 % Hide some
      |     param_vis(find(block_params == 'Neigh1')+NeighN:find(block_params == 'Neigh5')) = cellstr("off");
      | end
      | set_param(block,'MaskVisibilities',param_vis)
      mask DialogControl Container8 Prompt: Parameters
  ID3 : Subsystem  VariantControl=multi-agent  mask(gen_agent){ID=3, Leader=No leader, NeighN=2, Neigh1=2, Neigh2=4, Neigh3=0, Neigh4=0, Neigh5=0}
      mask prompts: ID "ID number"; Leader "Leader multi-agent"; NeighN "Number of neighbors"; Neigh1 "Neighbor 1"; Neigh2 "Neighbor 2"; Neigh3 "Neighbor 3"; Neigh4 "Neighbor 4"; Neigh5 "Neighbor 5"
      mask init: same as VFlexP_small/Grid/Dynamic/Secondary Control/MAS messages/ID1
      mask TypeOptions Leader: No leader | Leader
      mask TypeOptions NeighN: 1 | 2 | 3 | 4 | 5
      mask Callback NeighN:
      | block = gcb;
      | NeighN = str2double(get_param(block, 'NeighN'));
      | param_vis = get_param(block,'MaskVisibilities');
      | block_params = string(fieldnames(get_param(block, 'DialogParameters')));
      | param_vis(find(block_params == 'Neigh1'):find(block_params == 'Neigh5')) = cellstr("on");
      | if NeighN < 5 % Hide some
      |     param_vis(find(block_params == 'Neigh1')+NeighN:find(block_params == 'Neigh5')) = cellstr("off");
      | end
      | set_param(block,'MaskVisibilities',param_vis)
      mask DialogControl Container8 Prompt: Parameters
  ID4 : Subsystem  VariantControl=multi-agent  mask(gen_agent){ID=4, Leader=No leader, NeighN=2, Neigh1=3, Neigh2=5, Neigh3=0, Neigh4=0, Neigh5=0}
      mask prompts: ID "ID number"; Leader "Leader multi-agent"; NeighN "Number of neighbors"; Neigh1 "Neighbor 1"; Neigh2 "Neighbor 2"; Neigh3 "Neighbor 3"; Neigh4 "Neighbor 4"; Neigh5 "Neighbor 5"
      mask init: same as VFlexP_small/Grid/Dynamic/Secondary Control/MAS messages/ID1
      mask TypeOptions Leader: No leader | Leader
      mask TypeOptions NeighN: 1 | 2 | 3 | 4 | 5
      mask Callback NeighN:
      | block = gcb;
      | NeighN = str2double(get_param(block, 'NeighN'));
      | param_vis = get_param(block,'MaskVisibilities');
      | block_params = string(fieldnames(get_param(block, 'DialogParameters')));
      | param_vis(find(block_params == 'Neigh1'):find(block_params == 'Neigh5')) = cellstr("on");
      | if NeighN < 5 % Hide some
      |     param_vis(find(block_params == 'Neigh1')+NeighN:find(block_params == 'Neigh5')) = cellstr("off");
      | end
      | set_param(block,'MaskVisibilities',param_vis)
      mask DialogControl Container8 Prompt: Parameters
  ID5 : Subsystem  VariantControl=multi-agent  mask(gen_agent){ID=5, Leader=No leader, NeighN=2, Neigh1=4, Neigh2=6, Neigh3=0, Neigh4=0, Neigh5=0}
      mask prompts: ID "ID number"; Leader "Leader multi-agent"; NeighN "Number of neighbors"; Neigh1 "Neighbor 1"; Neigh2 "Neighbor 2"; Neigh3 "Neighbor 3"; Neigh4 "Neighbor 4"; Neigh5 "Neighbor 5"
      mask init: same as VFlexP_small/Grid/Dynamic/Secondary Control/MAS messages/ID1
      mask TypeOptions Leader: No leader | Leader
      mask TypeOptions NeighN: 1 | 2 | 3 | 4 | 5
      mask Callback NeighN:
      | block = gcb;
      | NeighN = str2double(get_param(block, 'NeighN'));
      | param_vis = get_param(block,'MaskVisibilities');
      | block_params = string(fieldnames(get_param(block, 'DialogParameters')));
      | param_vis(find(block_params == 'Neigh1'):find(block_params == 'Neigh5')) = cellstr("on");
      | if NeighN < 5 % Hide some
      |     param_vis(find(block_params == 'Neigh1')+NeighN:find(block_params == 'Neigh5')) = cellstr("off");
      | end
      | set_param(block,'MaskVisibilities',param_vis)
      mask DialogControl Container8 Prompt: Parameters
  ID6 : Subsystem  VariantControl=multi-agent  mask(gen_agent){ID=6, Leader=No leader, NeighN=2, Neigh1=5, Neigh2=7, Neigh3=0, Neigh4=0, Neigh5=0}
      mask prompts: ID "ID number"; Leader "Leader multi-agent"; NeighN "Number of neighbors"; Neigh1 "Neighbor 1"; Neigh2 "Neighbor 2"; Neigh3 "Neighbor 3"; Neigh4 "Neighbor 4"; Neigh5 "Neighbor 5"
      mask init: same as VFlexP_small/Grid/Dynamic/Secondary Control/MAS messages/ID1
      mask TypeOptions Leader: No leader | Leader
      mask TypeOptions NeighN: 1 | 2 | 3 | 4 | 5
      mask Callback NeighN:
      | block = gcb;
      | NeighN = str2double(get_param(block, 'NeighN'));
      | param_vis = get_param(block,'MaskVisibilities');
      | block_params = string(fieldnames(get_param(block, 'DialogParameters')));
      | param_vis(find(block_params == 'Neigh1'):find(block_params == 'Neigh5')) = cellstr("on");
      | if NeighN < 5 % Hide some
      |     param_vis(find(block_params == 'Neigh1')+NeighN:find(block_params == 'Neigh5')) = cellstr("off");
      | end
      | set_param(block,'MaskVisibilities',param_vis)
      mask DialogControl Container8 Prompt: Parameters
  ID7 : Subsystem  VariantControl=multi-agent  mask(gen_agent){ID=7, Leader=No leader, NeighN=2, Neigh1=6, Neigh2=1, Neigh3=0, Neigh4=0, Neigh5=0}
      mask prompts: ID "ID number"; Leader "Leader multi-agent"; NeighN "Number of neighbors"; Neigh1 "Neighbor 1"; Neigh2 "Neighbor 2"; Neigh3 "Neighbor 3"; Neigh4 "Neighbor 4"; Neigh5 "Neighbor 5"
      mask init: same as VFlexP_small/Grid/Dynamic/Secondary Control/MAS messages/ID1
      mask TypeOptions Leader: No leader | Leader
      mask TypeOptions NeighN: 1 | 2 | 3 | 4 | 5
      mask Callback NeighN:
      | block = gcb;
      | NeighN = str2double(get_param(block, 'NeighN'));
      | param_vis = get_param(block,'MaskVisibilities');
      | block_params = string(fieldnames(get_param(block, 'DialogParameters')));
      | param_vis(find(block_params == 'Neigh1'):find(block_params == 'Neigh5')) = cellstr("on");
      | if NeighN < 5 % Hide some
      |     param_vis(find(block_params == 'Neigh1')+NeighN:find(block_params == 'Neigh5')) = cellstr("off");
      | end
      | set_param(block,'MaskVisibilities',param_vis)
      mask DialogControl Container8 Prompt: Parameters
  Scope : Scope
      settings: ActiveDisplayYMinimum=0.09  ActiveDisplayYMaximum=0.11  DataLoggingVariableName=ScopeData2
  Scope1 : Scope
      settings: ActiveDisplayYMinimum=0.24945  ActiveDisplayYMaximum=4.0188
  Scope2 : Scope  NumInputPorts=2
      settings: ActiveDisplayYMinimum=9.9395  ActiveDisplayYMaximum=10.281  DataLoggingVariableName=ScopeData3
  Selector : Selector  NumberOfDimensions=2  InputPortWidth=3  IndexOptions=Index vector (dialog),Select all  Indices=1:6,1  OutputSizes=1,1
  Selector1 : Selector  NumberOfDimensions=2  InputPortWidth=3  IndexOptions=Index vector (dialog),Select all  Indices=7,1  OutputSizes=1,1
  Selector2 : Selector  NumberOfDimensions=2  InputPortWidth=3  IndexOptions=Index vector (dialog),Select all  Indices=8,1  OutputSizes=1,1
  Selector3 : Selector  NumberOfDimensions=2  InputPortWidth=3  IndexOptions=Index vector (dialog),Select all  Indices=2,1  OutputSizes=1,1
  Sum of Elements : Sum  Inputs=+
  Sum of Elements1 : Sum  Inputs=+
  concat : Concatenate  NumInputs=length(buses_lf)  Mode=Multidimensional array  ConcatenateDimension=2
  ref : Outport
  tag scope: Pmax=scoped, Snom=scoped, costs=scoped
  wires:
  Costs/1 -> [costs]
  Sum of Elements1/1 -> Scope2/2
  Sum of Elements/1 -> Scope2/1
  Selector3/1 -> Sum of Elements/1
  Selector2/1 -> Scope1/1
  Selector1/1 -> Scope/1, Sum of Elements1/1
  Selector/1 -> ref/1
  ID1/1(out) -> concat/1
  Constant1/1 -> [Snom]
  Constant2/1 -> [Pmax]
  elec/1 -> ID1/1(in), Selector3/1, ID2/1(in), ID3/1(in), ID4/1(in), ID5/1(in), ID6/1(in), ID7/1(in)
  concat/1 -> Selector/1, Selector1/1, Selector2/1
  ID2/1(out) -> concat/2
  ID3/1(out) -> concat/3
  ID4/1(out) -> concat/4
  ID5/1(out) -> concat/5
  ID6/1(out) -> concat/6
  ID7/1(out) -> concat/7

== system VFlexP_small/Grid/Dynamic/Tertiary Control/No TC ==
  elec : Inport
  connect_DGs : Inport  Port=2
  Constant : Constant  Value=[ones(1, length(buses_lf)); Ps_lf; v_buses_mod(buses_lf); Qs_lf]  VectorParams1D=off
  Matrix Concatenate2 : Concatenate  NumInputs=3  Mode=Multidimensional array
  Memory : Memory  InitialCondition=1
  Selector3 : Selector  NumberOfDimensions=2  InputPortWidth=3  IndexOptions=Index vector (dialog),Select all  Indices=6,1  OutputSizes=1,1
  ref : Outport
  wires:
  Memory/1 -> Matrix Concatenate2/3
  Constant/1 -> Matrix Concatenate2/1
  elec/1 -> Selector3/1
  Selector3/1 -> Memory/1
  [connect] -> Matrix Concatenate2/2
  connect_DGs/1 -> [connect]
  Matrix Concatenate2/1 -> ref/1

== system VFlexP_small/Grid/Dynamic/Tertiary Control/Scheduled ==
  elec : Inport
  connect_DGs : Inport  Port=2
  Constant1 : Constant  Value=v_buses_mod(buses_lf)  VectorParams1D=off
  Constant2 : Constant  Value=Qs_lf  VectorParams1D=off
  From Workspace : FromWorkspace  VariableName=[0 Ps_lf; Psche]  SampleTime=Psche(1,1)  Interpolate=off  OutputAfterFinalValue=Holding final value
  Matrix Concatenate2 : Concatenate  NumInputs=6  Mode=Multidimensional array
  One3 : Constant  Value=ones(1, length(buses_lf))  VectorParams1D=off  OutDataTypeStr=Inherit: Inherit via back propagation
  Selector6 : Selector  NumberOfDimensions=2  InputPortWidth=3  IndexOptions=Index vector (dialog),Select all  Indices=6,1  OutputSizes=1,1
  Transpose : Math  Operator=transpose
  ref : Outport
  wires:
  elec/1 -> Selector6/1
  connect_DGs/1 -> [connect]
  Matrix Concatenate2/1 -> ref/1
  Selector6/1 -> Matrix Concatenate2/6
  [connect] -> Matrix Concatenate2/5
  One3/1 -> Matrix Concatenate2/1
  Constant1/1 -> Matrix Concatenate2/3
  Constant2/1 -> Matrix Concatenate2/4
  From Workspace/1 -> Transpose/1
  Transpose/1 -> Matrix Concatenate2/2

== system VFlexP_small/Grid/Dynamic/iP/LPF ==
  In1 : Inport
  Gain : Gain  Gain=1e2
  I : Integrator  InitialCondition=[v_buses_mod; 0*v_buses_mod; 0*v_buses_mod]
  Sum4 : Sum  Inputs=|+-
  Out1 : Outport
  wires:
  Gain/1 -> I/1
  Sum4/1 -> Gain/1
  In1/1 -> Sum4/1
  I/1 -> Out1/1, Sum4/2

== system VFlexP_small/Grid/Dynamic/in_current/LPF ==
  In1 : Inport
  Gain : Gain  Gain=1e2
  I : Integrator  InitialCondition=[v_buses_mod; 0*v_buses_mod; 0*v_buses_mod]
  Sum4 : Sum  Inputs=|+-
  Out1 : Outport
  wires:
  Gain/1 -> I/1
  Sum4/1 -> Gain/1
  In1/1 -> Sum4/1
  I/1 -> Out1/1, Sum4/2

== system VFlexP_small/Grid/Loadflow/Generators/PC ==
  ioq : Inport
  iodi : Inport  Port=2
  omegaref : Inport  Port=3
  Eref : Inport  Port=4
  vodi : Inport  Port=5
  voq : Inport  Port=6
  Product{,1..3} (4 alike) : Product
  Sum : Sum  Inputs=|++
  Sum1 : Sum  Inputs=|-+
  Out1 : Outport
  Out2 : Outport  Port=2
  P_f : Outport  Port=3
  Q_f : Outport  Port=4
  wires:
  Sum1/1 -> Q_f/1
  Sum/1 -> P_f/1
  vodi/1 -> Product2/1, Product/1  "vod"
  Product/1 -> Sum/1
  Product1/1 -> Sum/2
  Product2/1 -> Sum1/1
  Product3/1 -> Sum1/2
  Eref/1 -> Out2/1  "Eref"
  omegaref/1 -> Out1/1  "omegaref"
  voq/1 -> Product1/1, Product3/1  "voq"
  iodi/1 -> Product3/2, Product/2  "iod"
  ioq/1 -> Product2/2, Product1/2  "ioq"

== system VFlexP_small/Grid/Loadflow/Generators/RL out ==
  note: 1) Add Subsystem or Model blocks as valid variant choices.
      | 2) You cannot connect blocks at this level. At simulation, connectivity is automatically
      | determined, based on the active variant and port name matching.
  v_in_d : Inport
  v_out_d : Inport  Port=2
  v_in_q : Inport  Port=3
  v_out_q : Inport  Port=4
  dynamic : Subsystem  VariantControl=dynamic
      settings: PortSchema="{\"entries\":[{\"content\":{\"sides\":[{\"content\":{\"connectorIds\":[\"In1\"]},\"type\":\"ConnectorPlacement.EquallySpacedRectSide\",\"uuid\":\"63966e24-f9e7-4b2d-b456-7f4ea5e3f230\"},{\"content\":{\"connectorIds\":[\"In2\",\"In3\",\"In4\",\"Out1\",\"Out2\"],\"side\":\"RIGHT\"},\"type\":\"ConnectorPlacement.EquallySpacedRectSide\",\"uuid\":\"ded6ef04-52fd-47df-8e49-cf16b827098d\"},{\"content\":{\"connectorIds\":[],\"side\":\"TOP\"},\"type\":\"ConnectorPlacement.EquallySpacedRectSide\",\"uuid\":\"f940a985-fa23-4968-ad44-1d76d0e20c6a\"}]},\"type\":\"ConnectorPlacement.EquallySpacedConnector\",\"uuid\":\"20f61d3c-9af2-4982-98ea-af4910e61c9c\"}],\"packageUris\":[\"http://schema.mathworks.com/mf0/Connector/R2020b\"],\"version\":\"1.0\"}"
  static : Subsystem  VariantControl=static
  static_omega : Subsystem  VariantControl=static_omega
  id : Outport
  iq : Outport  Port=2

== system VFlexP_small/Grid/Loadflow/Generators/Reference frame transform1 ==
  in_d : Inport
  theta : Inport  Port=2
  in_q : Inport  Port=3
  Complex to Real-Imag : ComplexToRealImag
  Cos : Trigonometry  SCDEnableBlockLinearizationSpecification=on  Operator=cos
  Product : Product
  Real-Imag to Complex : RealImagToComplex
  Real-Imag to Complex1 : RealImagToComplex
  Sin : Trigonometry  SCDEnableBlockLinearizationSpecification=on
  out_d : Outport
  out_q : Outport  Port=2
  wires:
  Complex to Real-Imag/2 -> out_q/1
  Real-Imag to Complex1/1 -> Product/1
  Real-Imag to Complex/1 -> Product/2
  Product/1 -> Complex to Real-Imag/1
  theta/1 -> Sin/1, Cos/1
  Cos/1 -> Real-Imag to Complex1/1
  Sin/1 -> Real-Imag to Complex1/2
  Complex to Real-Imag/1 -> out_d/1
  in_q/1 -> Real-Imag to Complex/2
  in_d/1 -> Real-Imag to Complex/1

== system VFlexP_small/Grid/Loadflow/Generators/Reference frame transform2 ==
  in_d : Inport
  theta : Inport  Port=2
  in_q : Inport  Port=3
  Complex to Real-Imag : ComplexToRealImag
  Cos : Trigonometry  SCDEnableBlockLinearizationSpecification=on  Operator=cos
  Product : Product
  Real-Imag to Complex : RealImagToComplex
  Real-Imag to Complex1 : RealImagToComplex
  Sin : Trigonometry  SCDEnableBlockLinearizationSpecification=on
  out_d : Outport
  out_q : Outport  Port=2
  wires:
  in_d/1 -> Real-Imag to Complex/1
  in_q/1 -> Real-Imag to Complex/2
  Complex to Real-Imag/1 -> out_d/1
  Sin/1 -> Real-Imag to Complex1/2
  Cos/1 -> Real-Imag to Complex1/1
  theta/1 -> Cos/1, Sin/1
  Product/1 -> Complex to Real-Imag/1
  Real-Imag to Complex/1 -> Product/2
  Real-Imag to Complex1/1 -> Product/1
  Complex to Real-Imag/2 -> out_q/1

== system VFlexP_small/Grid/Loadflow/Generators/Reference frame transform3 ==
  in_d : Inport
  theta : Inport  Port=2
  in_q : Inport  Port=3
  Complex to Real-Imag : ComplexToRealImag
  Cos : Trigonometry  SCDEnableBlockLinearizationSpecification=on  Operator=cos
  Product : Product
  Real-Imag to Complex : RealImagToComplex
  Real-Imag to Complex1 : RealImagToComplex
  Sin : Trigonometry  SCDEnableBlockLinearizationSpecification=on
  out_d : Outport
  out_q : Outport  Port=2
  wires:
  Complex to Real-Imag/2 -> out_q/1
  Real-Imag to Complex1/1 -> Product/1
  Real-Imag to Complex/1 -> Product/2
  Product/1 -> Complex to Real-Imag/1
  theta/1 -> Sin/1, Cos/1
  Cos/1 -> Real-Imag to Complex1/1
  Sin/1 -> Real-Imag to Complex1/2
  Complex to Real-Imag/1 -> out_d/1
  in_q/1 -> Real-Imag to Complex/2
  in_d/1 -> Real-Imag to Complex/1

== system VFlexP_small/Grid/Loadflow/Grid/Dynamic ==
  id_in : Inport
  iq_in : Inport  Port=2
  id_out : Inport  Port=3
  iq_out : Inport  Port=4
  Buses : Subsystem
  Complex to Real-Imag : ComplexToRealImag
  Gain : Gain  Gain=1./tap_lines.*(cos(shift_lines)-1i*sin(shift_lines))
  Lines : Subsystem
  Lines_From : MATLAB Function  TreatAsAtomicUnit=on
  Lines_From1 : MATLAB Function  TreatAsAtomicUnit=on
  Lines_To : MATLAB Function  TreatAsAtomicUnit=on
  Lines_To1 : MATLAB Function  TreatAsAtomicUnit=on
  One1 : Constant  Value=ones(1, length(From_buses))  VectorParams1D=off  OutDataTypeStr=Inherit: Inherit via back propagation
  Real-Imag to Complex : RealImagToComplex
  Selector4 : Selector  InputPortWidth=Nbuses  IndexOptions=Index vector (dialog)  Indices=From_buses  OutputSizes=1
  Selector5 : Selector  InputPortWidth=Nbuses  IndexOptions=Index vector (dialog)  Indices=From_buses  OutputSizes=1
  Selector6 : Selector  InputPortWidth=Nbuses  IndexOptions=Index vector (dialog)  Indices=To_buses  OutputSizes=1
  Selector7 : Selector  InputPortWidth=Nbuses  IndexOptions=Index vector (dialog)  Indices=To_buses  OutputSizes=1
  Sum{,1..3} (4 alike) : Sum  Inputs=|++
  vd : Outport
  vq : Outport  Port=2
  wires:
  Lines/2(iq) -> Real-Imag to Complex/2, Lines_To1/1(u)
  Lines_To/1(y) -> Sum/2
  One1/1 -> Lines/5(connected)
  Selector5/1 -> Lines/2(v_in_q)
  Lines/1(id) -> Real-Imag to Complex/1, Lines_To/1(u)
  Lines_From1/1(y) -> Sum3/2
  Sum2/1 -> Buses/2(i_d_out)
  Selector6/1 -> Lines/3(v_out_d)
  Lines_To1/1(y) -> Sum1/2
  Sum3/1 -> Buses/4(i_q_out)
  Sum/1 -> Buses/1(i_d_in)
  Selector7/1 -> Lines/4(v_out_q)
  Selector4/1 -> Lines/1(v_in_d)
  Buses/2(vq) -> Selector5/1, Selector7/1, vq/1  "voq"
  Buses/1(vd) -> vd/1, Selector6/1, Selector4/1  "vod"
  Lines_From/1(y) -> Sum2/2
  Sum1/1 -> Buses/3(i_q_in)
  id_in/1 -> Sum/1
  iq_in/1 -> Sum1/1
  id_out/1 -> Sum2/1
  iq_out/1 -> Sum3/1
  Gain/1 -> Complex to Real-Imag/1
  Real-Imag to Complex/1 -> Gain/1
  Complex to Real-Imag/1 -> Lines_From/1(u)
  Complex to Real-Imag/2 -> Lines_From1/1(u)

== system VFlexP_small/Grid/Loadflow/Grid/Static ==
  id_in : Inport
  iq_in : Inport  Port=2
  id_out : Inport  Port=3
  iq_out : Inport  Port=4
  Complex to Real-Imag : ComplexToRealImag
  Gain : Gain  Gain=iadmitt_matrix_noloads  Multiplication=Matrix(K*u)
  Real-Imag to Complex : RealImagToComplex
  Sum : Sum  Inputs=|+-
  Sum1 : Sum  Inputs=|+-
  Transpose : Math  Operator=transpose
  Transpose1 : Math  Operator=transpose
  vd : Outport
  vq : Outport  Port=2
  wires:
  Complex to Real-Imag/1 -> vd/1
  Sum1/1 -> Real-Imag to Complex/2  "iq1"
  Sum/1 -> Real-Imag to Complex/1  "id1"
  Complex to Real-Imag/2 -> vq/1
  Real-Imag to Complex/1 -> Transpose/1
  Gain/1 -> Transpose1/1
  id_in/1 -> Sum/1
  id_out/1 -> Sum/2
  iq_in/1 -> Sum1/1
  iq_out/1 -> Sum1/2
  Transpose/1 -> Gain/1
  Transpose1/1 -> Complex to Real-Imag/1

== system VFlexP_small/Grid/Loadflow/Loads/PQ ==
  v_in_d : Inport
  v_in_q : Inport  Port=2
  Constant : Constant  Value=Ploads(load_complexity_PF == 4)/Sb  VectorParams1D=off
  Constant1 : Constant  Value=Qloads(load_complexity_PF == 4)/Sb  VectorParams1D=off
  Divide : Product  Inputs=*/
  Divide1 : Product  Inputs=*/
  One1 : Constant  Value=eps  OutDataTypeStr=Inherit: Inherit via back propagation
  Product{,1..5} (6 alike) : Product
  Selector : Selector  InputPortWidth=length(Load_buses)  IndexOptions=Index vector (dialog)  Indices=find(load_complexity_PF == 4)  OutputSizes=1
  Selector1 : Selector  InputPortWidth=length(Load_buses)  IndexOptions=Index vector (dialog)  Indices=find(load_complexity_PF == 4)  OutputSizes=1
  Sum : Sum  Inputs=|++
  Sum1 : Sum  Inputs=|+-
  Sum4 : Sum  Inputs=|++
  Sum5 : Sum  Inputs=|++
  to_all_Loads : Subsystem
  to_all_Loads1 : Subsystem
  id : Outport
  iq : Outport  Port=2
  wires:
  Product1/1 -> Sum/2
  Product/1 -> Sum/1
  Constant/1 -> Product/1, Product2/1  "Prefnew"
  Product2/1 -> Sum1/1
  v_in_q/1 -> Selector1/1
  Product3/1 -> Sum1/2
  Product5/1 -> Sum4/2
  Constant1/1 -> Product3/1, Product1/2  "Qrefnew"
  Product4/1 -> Sum4/1
  Sum/1 -> Divide/1
  v_in_d/1 -> Selector/1
  Sum1/1 -> Divide1/1
  Sum5/1 -> Divide/2, Divide1/2
  Divide1/1 -> to_all_Loads1/1(In1)  "idref"
  Selector/1 -> Product4/1, Product4/2, Product/2, Product3/2
  to_all_Loads/1(Out1) -> id/1
  to_all_Loads1/1(Out1) -> iq/1
  Selector1/1 -> Product5/1, Product5/2, Product2/2, Product1/1
  Sum4/1 -> Sum5/1
  One1/1 -> Sum5/2
  Divide/1 -> to_all_Loads/1(In1)  "idref"
